simulink model "DashComm2015"  (Simulink 8.1)
settings: Solver=ode45  StartTime=0.0  StopTime=10.0  RelTol=1e-3
libraries: simulink x8
settings Model: Creator=Brian  LastModifiedBy=Brian
settings DataIOCC: SignalLoggingSaveFormat=Dataset
settings OptimizationCC: ExpressionDepthLimit=128
settings DebuggingCC: FcnCallInpInsideContextMsg=EnableAllAsError
settings GRTTargetCC: CombineOutputUpdateFcns=on  GRTInterface=off

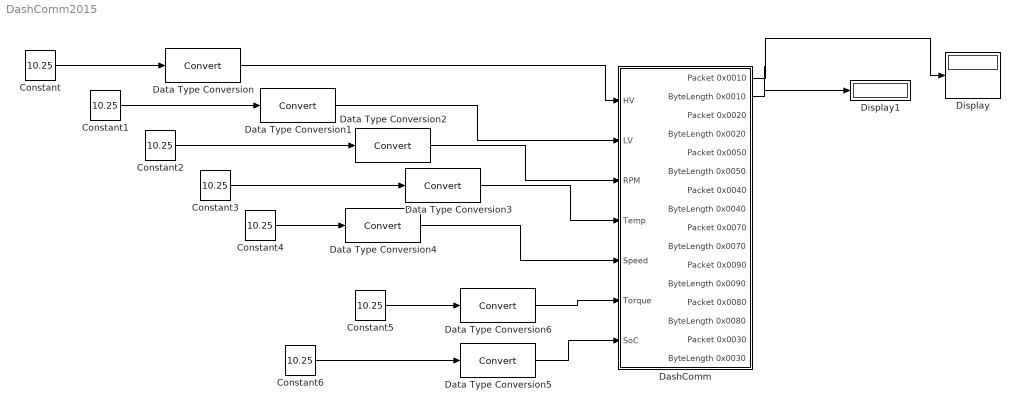
== system DashComm2015 ==
  Constant{,1..6} (7 alike) : Constant  Value=10.25
  DashComm : Subsystem
  Data Type Conversion{,1..6} (7 alike) : DataTypeConversion
  Display : Display
      settings: Format=hex (Stored Integer)
  Display1 : Display
      settings: Format=decimal (Stored Integer)
  wires:
  Constant/1 -> Data Type Conversion/1
  Constant1/1 -> Data Type Conversion1/1
  Constant2/1 -> Data Type Conversion2/1
  Constant3/1 -> Data Type Conversion3/1
  Constant4/1 -> Data Type Conversion4/1
  Constant6/1 -> Data Type Conversion5/1
  Constant5/1 -> Data Type Conversion6/1
  DashComm/1(Packet 0x0010) -> Display/1
  Data Type Conversion/1 -> DashComm/1(HV)
  Data Type Conversion1/1 -> DashComm/2(LV)
  Data Type Conversion2/1 -> DashComm/3(RPM)
  Data Type Conversion3/1 -> DashComm/4(Temp)
  Data Type Conversion4/1 -> DashComm/5(Speed)
  Data Type Conversion5/1 -> DashComm/7(SoC)
  Data Type Conversion6/1 -> DashComm/6(Torque)
  DashComm/2(ByteLength 0x0010) -> Display1/1

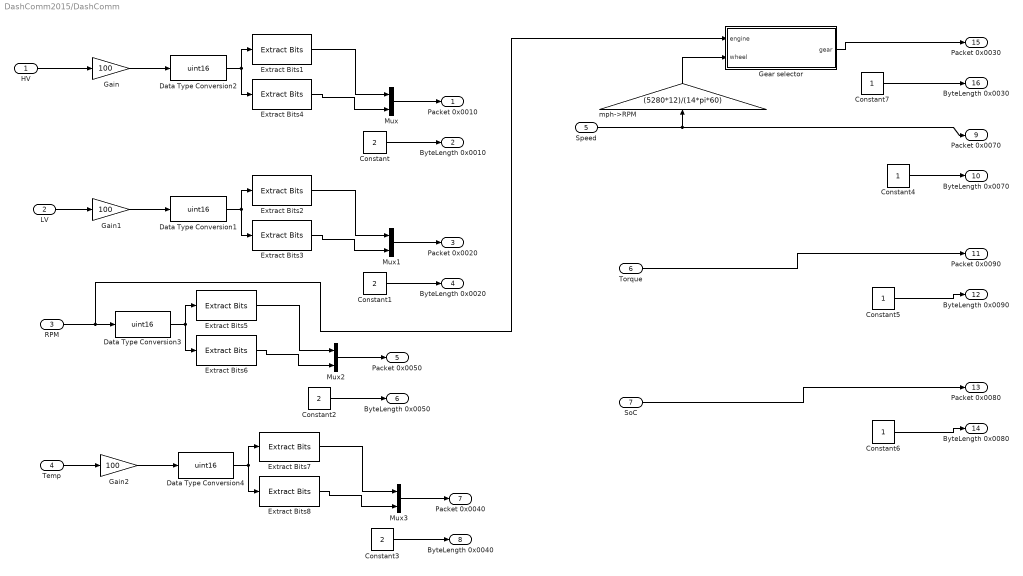
== system DashComm2015/DashComm ==
  HV : Inport  OutDataTypeStr=single
  LV : Inport  Port=2  OutDataTypeStr=single
  RPM : Inport  Port=3  OutDataTypeStr=uint16
  Temp : Inport  Port=4  OutDataTypeStr=uint8
  Speed : Inport  Port=5  OutDataTypeStr=uint8
  Torque : Inport  Port=6  OutDataTypeStr=int8
  SoC : Inport  Port=7  OutDataTypeStr=uint8
  Constant{,1..3} (4 alike) : Constant  Value=2  OutDataTypeStr=uint8
  Constant{4..7} (4 alike) : Constant  OutDataTypeStr=uint8
  Data Type Conversion{1..4} (4 alike) : DataTypeConversion  OutDataTypeStr=uint16  ConvertRealWorld=Stored Integer (SI)  LockScale=on
  Extract Bits{1..2,5,7} (4 alike) : simulink/Logic and Bit Operations/Extract Bits  bitsToExtract=Upper half  numBits=8  bitIdxRange=[0 7]  outScalingMode=Treat bit field as an integer
  Extract Bits{3..4,6,8} (4 alike) : simulink/Logic and Bit Operations/Extract Bits  bitsToExtract=Lower half  numBits=8  bitIdxRange=[0 7]  outScalingMode=Treat bit field as an integer
  Gain : Gain  Gain=100
  Gain1 : Gain  Gain=100
  Gain2 : Gain  Gain=100
  Gear selector : MATLAB Function  TreatAsAtomicUnit=on
  Mux{,1..3} (4 alike) : Mux  Inputs=2
  mph->RPM : Gain  Gain=(5280*12)/(14*pi*60)
  Packet 0x0010 : Outport
  ByteLength 0x0010 : Outport  Port=2  OutDataTypeStr=uint8
  Packet 0x0020 : Outport  Port=3
  ByteLength 0x0020 : Outport  Port=4  OutDataTypeStr=uint8
  Packet 0x0050 : Outport  Port=5
  ByteLength 0x0050 : Outport  Port=6  OutDataTypeStr=uint8
  Packet 0x0040 : Outport  Port=7
  ByteLength 0x0040 : Outport  Port=8  OutDataTypeStr=uint8
  Packet 0x0070 : Outport  Port=9
  ByteLength 0x0070 : Outport  Port=10  OutDataTypeStr=uint8
  Packet 0x0090 : Outport  Port=11
  ByteLength 0x0090 : Outport  Port=12  OutDataTypeStr=uint8
  Packet 0x0080 : Outport  Port=13
  ByteLength 0x0080 : Outport  Port=14  OutDataTypeStr=uint8
  Packet 0x0030 : Outport  Port=15
  ByteLength 0x0030 : Outport  Port=16  OutDataTypeStr=uint8
  wires:
  LV/1 -> Gain1/1
  Temp/1 -> Gain2/1
  Constant/1 -> ByteLength 0x0010/1
  Mux/1 -> Packet 0x0010/1
  Extract Bits4/1 -> Mux/2
  Extract Bits1/1 -> Mux/1
  HV/1 -> Gain/1
  Data Type Conversion2/1 -> Extract Bits4/1, Extract Bits1/1
  Gain/1 -> Data Type Conversion2/1
  Constant1/1 -> ByteLength 0x0020/1
  Mux1/1 -> Packet 0x0020/1
  Extract Bits3/1 -> Mux1/2
  Extract Bits2/1 -> Mux1/1
  Data Type Conversion1/1 -> Extract Bits3/1, Extract Bits2/1
  Gain1/1 -> Data Type Conversion1/1
  Constant2/1 -> ByteLength 0x0050/1
  Mux2/1 -> Packet 0x0050/1
  Extract Bits6/1 -> Mux2/2
  Extract Bits5/1 -> Mux2/1
  Data Type Conversion3/1 -> Extract Bits6/1, Extract Bits5/1
  Constant3/1 -> ByteLength 0x0040/1
  Mux3/1 -> Packet 0x0040/1
  Extract Bits8/1 -> Mux3/2
  Extract Bits7/1 -> Mux3/1
  Data Type Conversion4/1 -> Extract Bits8/1, Extract Bits7/1
  Gain2/1 -> Data Type Conversion4/1
  Speed/1 -> Packet 0x0070/1, mph->RPM/1
  Constant4/1 -> ByteLength 0x0070/1
  Torque/1 -> Packet 0x0090/1
  Constant5/1 -> ByteLength 0x0090/1
  SoC/1 -> Packet 0x0080/1
  Constant6/1 -> ByteLength 0x0080/1
  Constant7/1 -> ByteLength 0x0030/1
  Gear selector/1(gear) -> Packet 0x0030/1
  mph->RPM/1 -> Gear selector/2(wheel)
  RPM/1 -> Gear selector/1(engine), Data Type Conversion3/1

== matlab function DashComm/Gear selector ==
  data: engine input double; gear output double; wheel input double
function gear   = speedsToGear( engine,wheel )
    primary_gear = (24/73);
    gear1=13/32;
    gear2=16/32;
    gear3=17/28;
    gear4=19/26;
    gear5=21/25;
    sprockets=13/50;
    
    output_rpm = wheel;
    engine_rpm = engine;
    
    gear = 0;
    
    %calculates the engine speed for each gear based on the actual output
    engine_rpm1 = output_rpm/(primary_gear * sprockets * gear1);
    engine_rpm2 = output_rpm/(primary_gear * sprockets * gear2);
    engine_rpm3 = output_rpm/(primary_gear * sprockets * gear3);
    engine_rpm4 = output_rpm/(primary_gear * sprockets * gear4);
    engine_rpm5 = output_rpm/(primary_gear * sprockets * gear5);

    if engine_rpm1 <= engine_rpm + engine_rpm * .1 && engine_rpm1 >= engine_rpm - engine_rpm * .1
        gear = 1;
    end
    if engine_rpm2 <= engine_rpm + engine_rpm * .1 && engine_rpm2 >= engine_rpm - engine_rpm * .1
        gear = 2;
    end
    if engine_rpm3 <= engine_rpm + engine_rpm * .1 && engine_rpm3 >= engine_rpm - engine_rpm * .1
        gear = 3;
    end
    if engine_rpm4 <= engine_rpm + engine_rpm * .1 && engine_rpm4 >= engine_rpm - engine_rpm * .1
        gear = 4;
    end
    if engine_rpm5 <= engine_rpm + engine_rpm * .1 && engine_rpm5 >= engine_rpm - engine_rpm * .1
        gear = 5;
    end   
end
